simulink model "controller_model"  (R2026a)
settings: Solver=ode4  StopTime=1.0  FixedStep=0.001
undefined symbols (not defined in the file): Ts
settings Model: Creator=anh  LastModifiedBy=anh
settings DataIOCC: ExternalInput=p_drv_in, lam_in, v_veh_in

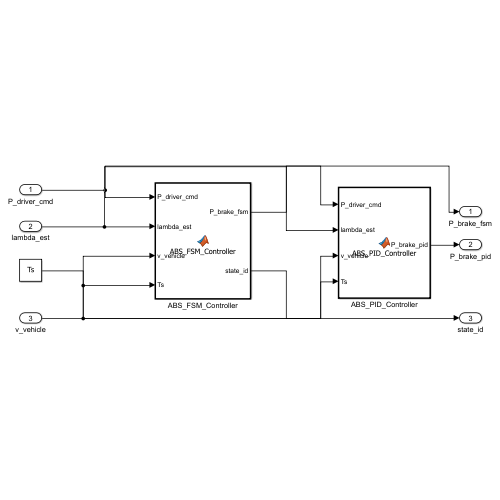
[thumbnail: Simulink's stored preview of the top-level diagram]
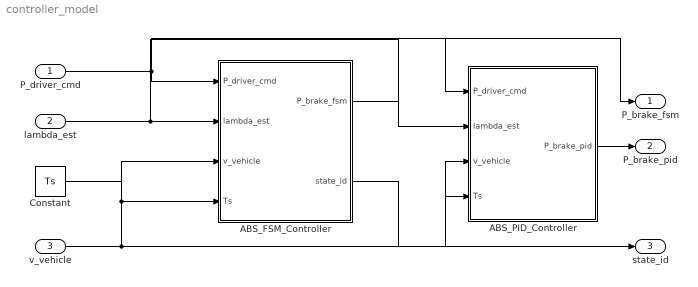
== system controller_model ==
  P_driver_cmd : Inport
  lambda_est : Inport  Port=2
  v_vehicle : Inport  Port=3
  ABS_FSM_Controller : MATLAB Function  TreatAsAtomicUnit=on
  ABS_PID_Controller : MATLAB Function  TreatAsAtomicUnit=on
  Constant : Constant  Value=Ts
  P_brake_fsm : Outport
  P_brake_pid : Outport  Port=2
  state_id : Outport  Port=3
  wires:
  Constant/1 -> ABS_FSM_Controller/4(Ts), ABS_PID_Controller/4(Ts)
  P_driver_cmd/1 -> ABS_FSM_Controller/1(P_driver_cmd), ABS_PID_Controller/1(P_driver_cmd)
  lambda_est/1 -> ABS_PID_Controller/2(lambda_est), ABS_FSM_Controller/2(lambda_est)
  v_vehicle/1 -> ABS_FSM_Controller/3(v_vehicle), ABS_PID_Controller/3(v_vehicle)
  ABS_FSM_Controller/1(P_brake_fsm) -> P_brake_fsm/1
  ABS_FSM_Controller/2(state_id) -> state_id/1
  ABS_PID_Controller/1(P_brake_pid) -> P_brake_pid/1

== matlab function controller_model/ABS_PID_Controller ==
  data: P_driver_cmd input; P_brake_pid output; lambda_est input; v_vehicle input; Ts input
function P_brake_pid = ABS_PID_Controller(P_driver_cmd, lambda_est, v_vehicle, Ts)
% ABS_PID_CONTROLLER Bộ điều khiển PID bám tỉ số trượt mục tiêu (lambda_target = 0.20)

persistent e_int e_prev

if isempty(e_int)
    e_int = 0.0;
    e_prev = 0.0;
end

% Tắt ABS khi tốc độ quá thấp (v < 5 m/s)
if v_vehicle < 5.0
    P_brake_pid = P_driver_cmd;
    e_int = 0.0;
    e_prev = 0.0;
    return;
end

% Sai lệch tỉ số trượt (ngược dấu vì trượt tăng -> cần giảm áp)
lambda_target = 0.20;
error = lambda_est - lambda_target;

% Hệ số PID tuned
Kp = 400.0;
Ki = 1000.0;
Kd = 15.0;

% Tích phân có Anti-Windup Clamping [-50, 50]
e_int = e_int + error * Ts;
e_int = max(-50.0, min(50.0, e_int));

% Đạo hàm
e_der = (error - e_prev) / Ts;
e_prev = error;

% Tín hiệu giảm áp suất delta P
delta_P = Kp * error + Ki * e_int + Kd * e_der;

% Áp suất phanh PID
P_raw = P_driver_cmd - delta_P;

% Giới hạn an toàn thủy lực [0, P_driver_cmd]
P_brake_pid = max(0.0, min(P_driver_cmd, P_raw));
end

== matlab function controller_model/ABS_FSM_Controller ==
  data: P_driver_cmd input; P_brake_fsm output; lambda_est input; v_vehicle input; Ts input; state_id output
function [P_brake_fsm, state_id] = ABS_FSM_Controller(P_driver_cmd, lambda_est, v_vehicle, Ts)
% ABS_FSM_CONTROLLER Máy trạng thái hữu hạn (FSM) điều khiển phanh ABS Bang-Bang
%
% States:
%   1: NORMAL - Phanh bình thường (P = P_driver_cmd)
%   2: BUILD  - Tăng áp suất phanh (+800 bar/s)
%   3: HOLD   - Giữ nguyên áp suất phanh (dP/dt = 0)
%   4: DUMP   - Xả áp suất phanh nhanh (-1200 bar/s)

persistent current_state P_internal

if isempty(current_state)
    current_state = 1; % Mặc định NORMAL
    P_internal = 0.0;
end

% 1. Cắt an toàn ở tốc độ thấp (v < 5 m/s -> Tắt ABS, trả quyền phanh tự nhiên)
if v_vehicle < 5.0
    current_state = 1;
end

% 2. Chuyển trạng thái máy FSM
switch current_state
    case 1 % NORMAL
        P_internal = P_driver_cmd;
        if (v_vehicle >= 5.0) && (lambda_est > 0.15)
            current_state = 2; % Sang BUILD
        end

    case 2 % BUILD (+800 bar/s)
        P_internal = P_internal + 800.0 * Ts;
        if lambda_est >= 0.20
            current_state = 3; % Sang HOLD
        end

    case 3 % HOLD (dP/dt = 0)
        if lambda_est >= 0.25
            current_state = 4; % Sang DUMP
        elseif lambda_est < 0.18
            current_state = 2; % Về BUILD
        end

    case 4 % DUMP (-1200 bar/s)
        P_internal = P_internal - 1200.0 * Ts;
        if lambda_est <= 0.20
            current_state = 3; % Về HOLD
        end
end

% 3. Khống chế giới hạn an toàn thủy lực [0, P_driver_cmd]
P_brake_fsm = max(0.0, min(P_driver_cmd, P_internal));
state_id = double(current_state);
end
